simulink library "dac20"  (Simulink 8.6)
settings: Solver=ode45  SolverMode=SingleTasking  StartTime=0.0  StopTime=10.0  RelTol=1e-3
settings Model: Creator=rolf  LastModifiedBy=rolf

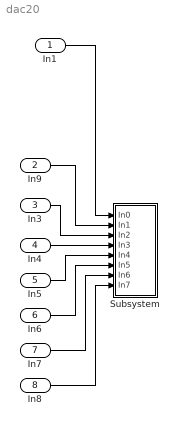
== system dac20 ==
  In1 : Inport
  In9 : Inport  Port=2
  In3 : Inport  Port=3
  In4 : Inport  Port=4
  In5 : Inport  Port=5
  In6 : Inport  Port=6
  In7 : Inport  Port=7
  In8 : Inport  Port=8
  Subsystem : Subsystem
  wires:
  In1/1 -> Subsystem/1(In0)
  In3/1 -> Subsystem/3(In2)
  In4/1 -> Subsystem/4(In3)
  In5/1 -> Subsystem/5(In4)
  In6/1 -> Subsystem/6(In5)
  In7/1 -> Subsystem/7(In6)
  In8/1 -> Subsystem/8(In7)
  In9/1 -> Subsystem/2(In1)

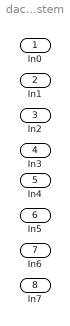
== system dac20/Subsystem ==
  In0 : Inport
  In1 : Inport  Port=2
  In2 : Inport  Port=3
  In3 : Inport  Port=4
  In4 : Inport  Port=5
  In5 : Inport  Port=6
  In6 : Inport  Port=7
  In7 : Inport  Port=8
